simulink model "Hector"  (R2023b)
settings: Solver=daessc  StartTime=0.0  StopTime=1  FixedStep=0.001  MaxStep=1e-3  RelTol=1e-2
model workspace (MATLAB code in the model file):
  | %% World Plane
  | plane_x = 20;
  | plane_y = 2;
  | plane_z = 0.05;
  | 
  | %% motor
  | %A1
  | motor_com = [0, -0.02,0];
  | motor_com_mirror = [0, 0.02,0];
  | 
  | motor_I = [0.00048,0.00071,0.00048];
  | motor_mass = 0.605;
  | 
  | %% Body
  | % Inertial
  | body_com_x = 0.0;
  | body_com_y = 0.0;
  | body_com_z = -0.0;
  | body_mass = 5.75;
  | body_ixx = 44350*1e-6;
  | body_ixy = 0.0;
  | body_ixz = 0.0;
  | body_iyy = 53149*1e-6;
  | body_iyz = 0.0;
  | body_izz = 21390*1e-6;
  | 
  | %% Hip 1
  | % joint
  | hip1_offset_x =0.0;
  | hip1_offset_y = 0.047;
  | hip1_offset_z = 0.1265;
  | % hip1_max = 15;
  | % hip1_min = -15;
  | hip1_velocity_max = 21;
  | hip1_torque_max = 33.5;
  | % Inertial
  | hip1_com_x = 0.0268;
  | hip1_com_y = -0.00315;
  | hip1_com_z = -0.0272;
  | hip1_mass = 0.173;
  | hip1_ixx = 0.00022;
  | hip1_ixy = 0.0;
  | hip1_ixz = 0.0;
  | hip1_iyy = 0.00024;
  | hip1_iyz = 0.0;
  | hip1_izz = 0.00016;
  | 
  | %% Hip 2
  | % joint
  | hip2_offset_x =0.053;
  | hip2_offset_y = 0.0185;
  | hip2_offset_z = 0.071;
  | % hip2_max = 15;
  | % hip2_min = -15;
  | hip2_velocity_max = 21;
  | hip2_torque_max = 33.5;
  | % Inertial
  | hip2_com_x = -0.0308;
  | hip2_com_y = -0.00942;
  | hip2_com_z = 0.0;
  | hip2_mass = 0.0722;
  | hip2_ixx = 0.0000422;
  | hip2_ixy = 0.0;
  | hip2_ixz = 0.0;
  | hip2_iyy = 0.000120;
  | hip2_iyz = 0.0;
  | hip2_izz = 0.0000708;
  | 
  | %% Thigh
  | % joint
  | thigh_offset_x =-0.06;
  | thigh_offset_y = 0.004;
  | thigh_offset_z = 0.0;
  | % thigh_max = 130;
  | % thigh_min = -45;
  | thigh_velocity_max = 21;
  | thigh_torque_max = 33.5;
  | % Inertial
  | thigh_com_x = -0.00143;
  | thigh_com_y = -0.02106;
  | thigh_com_z = -0.06115;
  | thigh_mass = 0.397;
  | thigh_ixx = 0.00197;
  | thigh_ixy = 0.0;
  | thigh_ixz = 0.0;
  | thigh_iyy = 0.00218;
  | thigh_iyz = 0.0;
  | thigh_izz = 0.00033;
  | 
  | ankle_motor_offset_x = 0;
  | ankle_motor_offset_y = 0.039;
  | ankle_motor_offset_z = 0;
  | 
  | knee_motor_offset_x = 0;
  | knee_motor_offset_y = 0.039;
  | knee_motor_offset_z = -0.095;
  | 
  | %% Calf
  | % joint
  | calf_offset_x = 0.0;
  | calf_offset_y = 0.003;
  | calf_offset_z = -0.22;
  | % calf_max = 0;
  | % calf_min = -135;
  | % knee_max = 0;
  | % knee_min = -160;
  | calf_velocity_max = 14*1.5;
  | calf_torque_max = 51;
  | % Inertial
  | calf_com_x = 0.00165;
  | calf_com_y = -0.01117;
  | calf_com_z = -0.06438;
  | calf_mass = 0.136;
  | calf_ixx = 0.00071;
  | calf_ixy = 0.0;
  | calf_ixz = 0.0;
  | calf_iyy = 0.00072;
  | calf_iyz = 0.0;
  | calf_izz = 0.00002;
  | 
  | %% Toe
  | % joint
  | toe_offset_x = 0.0;
  | toe_offset_y = 0.011;
  | toe_offset_z = -0.22;
  | % toe_max = 60;
  | % toe_min = -60;
  | toe_velocity_max = 21;
  | toe_torque_max = 33.5;
  | % Inertial
  | toe_com_x = 0.00239;
  | toe_com_y = 0.00002;
  | toe_com_z = -0.02261;
  | toe_mass = 0.08425;
  | toe_ixx = 0.00001;
  | toe_ixy = 0.0;
  | toe_ixz = 0.0;
  | toe_iyy = 0.00011;
  | toe_iyz = 0.0;
  | toe_izz = 0.00011;
  | %% Contact
  | contact_front = 0.091;
  | contact_rear = -0.061;
  | contact_right = 0.026;
  | contact_left = 0.01;
  | contact_z = 0.039;
  | 
  | %%
  | %dorito
  | dorito_offset_x = 0;
  | dorito_offset_y = 0.012;
  | dorito_offset_z = 0;
  | 
  | dorito_lower_connection = [0.034 0 -0.044];
  | dorito_upper_connection = [0.034 0 0.021];
  | 
  | linkage_mass = 0.051;
  | linkage_com = [0 0 -0.11];
  | linkage_I = [0.00001 0.00002 0.00002];
  | %% Arms
  | shoulder_com_x = 0;
  | shoulder_com_y = 0;
  | shoulder_com_z = 0;
  | shoulder_mass = 0.835;
  | % shoulder_mass = 0.05;
  | shoulder_ixx = 920*1e-6;
  | shoulder_ixy = 0.0;
  | shoulder_ixz = 0.0;
  | shoulder_iyy = 270*1e-6;
  | shoulder_iyz = 0.0;
  | shoulder_izz = 499*1e-6;
  | 
  | upperarm_com_x = 0;
  | upperarm_com_y = 0;
  | upperarm_com_z = 0;
  | upperarm_mass = 1.35;
  | % upperarm_mass = 0.05;
  | upperarm_ixx = 1200*1e-6;
  | upperarm_ixy = 0.0;
  | upperarm_ixz = 0.0;
  | upperarm_iyy = 1170*1e-6;
  | upperarm_iyz = 0.0;
  | upperarm_izz = 729*1e-6;
  | 
  | forearm_com_x = 0;
  | forearm_com_y = 0;
  | forearm_com_z = -0.10;
  | forearm_mass = 0.53;
  | % forearm_mass = 0.03;
  | forearm_ixx = 427*1e-6;
  | forearm_ixy = 0.0;
  | forearm_ixz = 0.0;
  | forearm_iyy = 466*1e-6;
  | forearm_iyz = 0.0;
  | forearm_izz = 72*1e-6;
values from neighbouring files (symbols this model uses):
  body_v0 = [0 0 0]    [Initiate_Simulation.m]
  body_z0 = 0.55    [Initiate_Simulation.m]
  dt_MPC = gaitcycle/10    (= 0.04)    [Initiate_Simulation.m]
  N = 5000    [Initiate_Simulation.m]
  shoulderx_max = 90    [Initiate_Simulation.m]
  shoulderx_min = -15    [Initiate_Simulation.m]
  shoulderx_q0 = 0    [Initiate_Simulation.m]
undefined symbols (not defined in the file or in its folder): AssignMPCStage, sigbuilder_block, X, Y, Z
libraries: sm_lib x169, nesl_utility x95, dspindex x1, simulink x1
(part 5 of 7)

== system Hector/Hector/Left Leg/calf ==
  Joint : Inport
  Knee Joint : Subsystem
      settings: PortSchema="{\"entries\":[{\"content\":{\"sides\":[{\"content\":{\"connectorIds\":[\"LConn1\",\"In1\"]},\"type\":\"ConnectorPlacement.EquallySpacedRectSide\",\"uuid\":\"fe1bafd1-c1a5-4148-b465-5de294b235b8\"},{\"content\":{\"connectorIds\":[\"RConn1\",\"Out1\",\"Out2\",\"Out3\"],\"side\":\"RIGHT\"},\"type\":\"ConnectorPlacement.EquallySpacedRectSide\",\"uuid\":\"cbba8e06-0841-4611-b08d-047237296da9\"},{\"content\":{\"connectorIds\":[],\"side\":\"TOP\"},\"type\":\"ConnectorPlacement.EquallySpacedRectSide\",\"uuid\":\"b5035594-e8f7-4741-b410-9cfafd0751b0\"}]},\"type\":\"ConnectorPlacement.EquallySpacedConnector\",\"uuid\":\"2233606c-74e6-45bf-8a73-f401921fd730\"}],\"packageUris\":[\"http://schema.mathworks.com/mf0/Connector/R2020b\"],\"version\":\"1.0\"}"
  Rigid Transform4 : sm_lib/Frames and Transforms/Rigid Transform  TranslationMethod=None  TranslationStandardOffset=0  TranslationStandardOffsetUnits=m  TranslationStandardAxis=+Z  TranslationCartesianOffset=[0 0 0]  TranslationCartesianOffsetUnits=m  TranslationROffset=0  TranslationROffsetUnits=m  TranslationZOffset=0  TranslationZOffsetUnits=m  TranslationThetaOffset=0  TranslationThetaOffsetUnits=deg  RotationMethod=StandardAxis  RotationAngleUnits=deg  RotationStandardAxis=-X  RotationAngle=90  RotationArbitraryAxis=[0 0 1]  FollAlignAxisA=+X  BaseAlignAxisA=+Y  FollAlignAxisB=+Y  BaseAlignAxisB=+Z  RotationSequenceAxes=FollowerAxes  RotationSequence=XYX  RotationSequenceAngles=[0 0 0]  RotationSequenceAnglesUnits=deg  RotationMatrix=[1 0 0; 0 1 0; 0 0 1]  Quaternion=[1 0 0 0]
  Rigid Transform5 : sm_lib/Frames and Transforms/Rigid Transform  TranslationMethod=None  TranslationStandardOffset=0  TranslationStandardOffsetUnits=m  TranslationStandardAxis=+Z  TranslationCartesianOffset=[0 0 0]  TranslationCartesianOffsetUnits=m  TranslationROffset=0  TranslationROffsetUnits=m  TranslationZOffset=0  TranslationZOffsetUnits=m  TranslationThetaOffset=0  TranslationThetaOffsetUnits=deg  RotationMethod=StandardAxis  RotationAngleUnits=deg  RotationStandardAxis=+X  RotationAngle=90  RotationArbitraryAxis=[0 0 1]  FollAlignAxisA=+X  BaseAlignAxisA=+Y  FollAlignAxisB=+Y  BaseAlignAxisB=+Z  RotationSequenceAxes=FollowerAxes  RotationSequence=XYX  RotationSequenceAngles=[0 0 0]  RotationSequenceAnglesUnits=deg  RotationMatrix=[1 0 0; 0 1 0; 0 0 1]  Quaternion=[1 0 0 0]
  calf : sm_lib/Body Elements/File Solid  ExtGeomFileName=STL files\L_calf.STL  UnitType=Custom  ExtGeomFileUnits=m  StepReaderType=HEX  ExportConvexHullGeometry=off  InertiaType=Custom  Mass=calf_mass  MassUnits=kg  CenterOfMass=[calf_com_x -calf_com_y calf_com_z]  CenterOfMassUnits=m  MomentsOfInertia=[calf_ixx calf_iyy calf_izz]  MomentsOfInertiaUnits=kg*m^2  ProductsOfInertia=[0 0 0]  ProductsOfInertiaUnits=kg*m^2  BasedOnType=Density  Density=1000  DensityUnits=kg/m^3  DoExposeReferenceFrame=on  SerializedFrames=<Frames/>  GraphicType=FromGeometry  MarkerShape=Sphere  MarkerSize=10  GraphicVisPropType=AdvancedVisualProperties  GraphicDiffuseColor=[0.9 0.9 0.9]  GraphicSpecularColor=[0.7 0.7 0.7 1.0]  GraphicAmbientColor=[0.35 0.35 0.35 1.0]  GraphicEmissiveColor=[0.0 0.0 0.0 1.0]  GraphicShininess=5  GraphicOpacity=1.0
  B : PMIOPort  Side=Left
  Conn2 : PMIOPort  Port=2  Side=Right
  Sensor : Outport
  knee_angle : Outport  Port=2
  knee_angle_speed : Outport  Port=3
  wires:
  Knee Joint/2(knee_angle) -> knee_angle/1
  Knee Joint/3(knee_angle_speed) -> knee_angle_speed/1
  Knee Joint/1(Sensor) -> Sensor/1
  Joint/1 -> Knee Joint/1(Joint)
  connections:
  calf/RConn1 -- Rigid Transform4/LConn1
  Knee Joint/LConn1 -- B/RConn1
  Rigid Transform5/LConn1 -- Knee Joint/RConn1 -- Rigid Transform4/RConn1
  Rigid Transform5/RConn1 -- Conn2/RConn1

== system Hector/Hector/Left Leg/foot ==
  input : Inport
  Ankle Joint : Subsystem
      settings: PortSchema="{\"entries\":[{\"content\":{\"sides\":[{\"content\":{\"connectorIds\":[\"LConn1\",\"In1\"]},\"type\":\"ConnectorPlacement.EquallySpacedRectSide\",\"uuid\":\"d1094410-d7e2-420f-9299-c6db7682fd14\"},{\"content\":{\"connectorIds\":[\"RConn1\",\"Out1\"],\"side\":\"RIGHT\"},\"type\":\"ConnectorPlacement.EquallySpacedRectSide\",\"uuid\":\"17ca1f8d-2ad9-48dc-a054-4cdfe8b39b0e\"},{\"content\":{\"side\":\"TOP\"},\"type\":\"ConnectorPlacement.EquallySpacedRectSide\",\"uuid\":\"c0a1fb68-cc05-4666-9aff-395b76c49866\"}]},\"type\":\"ConnectorPlacement.EquallySpacedConnector\",\"uuid\":\"a0ca8f3e-9cc5-4e2d-aebb-075ea702600d\"}],\"packageUris\":[\"http://schema.mathworks.com/mf0/Connector/R2020b\"],\"version\":\"1.0\"}"
  Foot : sm_lib/Body Elements/File Solid  ExtGeomFileName=STL files\L_foot.STL  UnitType=Custom  ExtGeomFileUnits=m  StepReaderType=HEX  ExportConvexHullGeometry=off  InertiaType=Custom  Mass=toe_mass  MassUnits=kg  CenterOfMass=[toe_com_x toe_com_y toe_com_z]  CenterOfMassUnits=m  MomentsOfInertia=[toe_ixx toe_iyy toe_izz]  MomentsOfInertiaUnits=kg*m^2  ProductsOfInertia=[0 0 0]  ProductsOfInertiaUnits=kg*m^2  BasedOnType=Density  Density=1000  DensityUnits=kg/m^3  DoExposeReferenceFrame=on  SerializedFrames=<Frames/>  GraphicType=FromGeometry  MarkerShape=Sphere  MarkerSize=10  GraphicVisPropType=AdvancedVisualProperties  GraphicDiffuseColor=[0.9 0.9 0.9]  GraphicSpecularColor=[0.7 0.7 0.7 1.0]  GraphicAmbientColor=[0.35 0.35 0.35 1.0]  GraphicEmissiveColor=[0.0 0.0 0.0 1.0]  GraphicShininess=5  GraphicOpacity=1.0
  Rigid Transform1 : sm_lib/Frames and Transforms/Rigid Transform  TranslationMethod=Cartesian  TranslationStandardOffset=0  TranslationStandardOffsetUnits=m  TranslationStandardAxis=+Z  TranslationCartesianOffset=[0 0.01 0]  TranslationCartesianOffsetUnits=m  TranslationROffset=0  TranslationROffsetUnits=m  TranslationZOffset=0  TranslationZOffsetUnits=m  TranslationThetaOffset=0  TranslationThetaOffsetUnits=deg  RotationMethod=None  RotationAngleUnits=deg  RotationStandardAxis=-X  RotationAngle=90  RotationArbitraryAxis=[0 0 1]  FollAlignAxisA=+X  BaseAlignAxisA=+Y  FollAlignAxisB=+Y  BaseAlignAxisB=+Z  RotationSequenceAxes=FollowerAxes  RotationSequence=XYX  RotationSequenceAngles=[0 0 0]  RotationSequenceAnglesUnits=deg  RotationMatrix=[1 0 0; 0 1 0; 0 0 1]  Quaternion=[1 0 0 0]
  Rigid Transform6 : sm_lib/Frames and Transforms/Rigid Transform  TranslationMethod=None  TranslationStandardOffset=0  TranslationStandardOffsetUnits=m  TranslationStandardAxis=+Z  TranslationCartesianOffset=[0 0 0]  TranslationCartesianOffsetUnits=m  TranslationROffset=0  TranslationROffsetUnits=m  TranslationZOffset=0  TranslationZOffsetUnits=m  TranslationThetaOffset=0  TranslationThetaOffsetUnits=deg  RotationMethod=StandardAxis  RotationAngleUnits=deg  RotationStandardAxis=-X  RotationAngle=90  RotationArbitraryAxis=[0 0 1]  FollAlignAxisA=+X  BaseAlignAxisA=+Y  FollAlignAxisB=+Y  BaseAlignAxisB=+Z  RotationSequenceAxes=FollowerAxes  RotationSequence=XYX  RotationSequenceAngles=[0 0 0]  RotationSequenceAnglesUnits=deg  RotationMatrix=[1 0 0; 0 1 0; 0 0 1]  Quaternion=[1 0 0 0]
  B : PMIOPort  Side=Left
  Conn4 : PMIOPort  Port=2  Side=Right
  F : PMIOPort  Port=3  Side=Right
  sensor : Outport
  wires:
  input/1 -> Ankle Joint/1(input)
  Ankle Joint/1(sensor) -> sensor/1
  connections:
  Rigid Transform6/RConn1 -- Ankle Joint/RConn1
  Ankle Joint/LConn1 -- B/RConn1
  Rigid Transform6/LConn1 -- Conn4/RConn1 -- Rigid Transform1/RConn1 -- F/RConn1
  Rigid Transform1/LConn1 -- Foot/RConn1

== system Hector/Hector/Left Leg/hip location sensor ==
  Bus Creator : BusCreator  Inputs=3
  PS-Simulink Converter : nesl_utility/PS-Simulink Converter  PhysicalDomain=network_engine_domain  SubClassName=ps_output  LeftPortType=input  RightPortType=output  PseudoPeriodic=off  Frequencies=[]  VectorFormat=1-D array  Unit=inherit  AffineConversion=off
  PS-Simulink Converter1 : nesl_utility/PS-Simulink Converter  PhysicalDomain=network_engine_domain  SubClassName=ps_output  LeftPortType=input  RightPortType=output  PseudoPeriodic=off  Frequencies=[]  VectorFormat=1-D array  Unit=inherit  AffineConversion=off
  PS-Simulink Converter2 : nesl_utility/PS-Simulink Converter  PhysicalDomain=network_engine_domain  SubClassName=ps_output  LeftPortType=input  RightPortType=output  PseudoPeriodic=off  Frequencies=[]  VectorFormat=1-D array  Unit=inherit  AffineConversion=off
  Transform Sensor : sm_lib/Frames and Transforms/Transform Sensor  MeasurementFrame=World  RotationSequence=XYX  SenseAngle=off  SenseAxis=off  SenseQ=off  SenseR=off  SenseRotationSequence=off  SenseOmegaX=off  SenseOmegaY=off  SenseOmegaZ=off  SenseOmega=off  SenseQDot=off  SenseRDot=off  SenseRotationSequenceDot=off  SenseAlphaX=off  SenseAlphaY=off  SenseAlphaZ=off  SenseAlpha=off  SenseQDDot=off  SenseRDDot=off  SenseX=on  SenseY=on  SenseZ=on  SenseXYZ=off  SenseRad=off  SenseAzim=off  SenseDist=off  SenseInc=off  SenseXDot=off  SenseYDot=off  SenseZDot=off  SenseXYZDot=off  SenseRadDot=off  SenseAzimDot=off  SenseDistDot=off  SenseIncDot=off  SenseXDDot=off  SenseYDDot=off  SenseZDDot=off  SenseXYZDDot=off  SenseRadDDot=off  SenseAzimDDot=off  SenseDistDDot=off  SenseIncDDot=off
  World Frame : sm_lib/Frames and Transforms/World Frame
  R : PMIOPort  Side=Right
  hip_location : Outport
  wires:
  PS-Simulink Converter1/1 -> Bus Creator/2  "y"
  PS-Simulink Converter/1 -> Bus Creator/1  "x"
  PS-Simulink Converter2/1 -> Bus Creator/3  "z"
  Bus Creator/1 -> hip_location/1
  connections:
  PS-Simulink Converter2/LConn1 -- Transform Sensor/RConn4
  PS-Simulink Converter/LConn1 -- Transform Sensor/RConn2
  World Frame/RConn1 -- Transform Sensor/LConn1
  PS-Simulink Converter1/LConn1 -- Transform Sensor/RConn3
  Transform Sensor/RConn1 -- R/RConn1

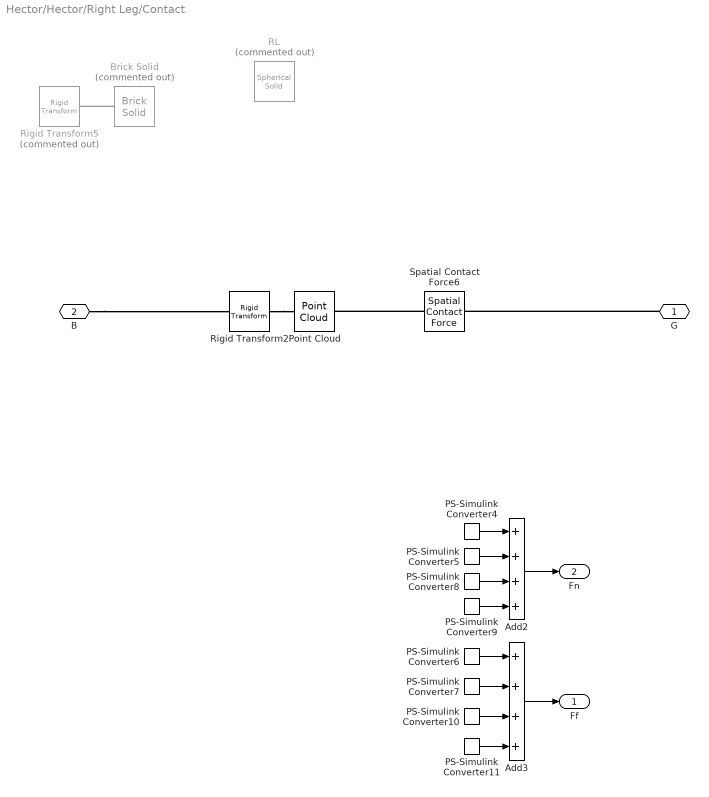
== system Hector/Hector/Right Leg/Contact ==
  Add2 : Sum  Inputs=++++
  Add3 : Sum  Inputs=++++
  Brick Solid : sm_lib/Body Elements/Brick Solid  Commented=on  GraphicAmbientColor=[0.15 0.15 0.15 1.0]  BasedOnType=Density  BrickDimensions=[0.16 0.02 0.0001]  BrickDimensionsUnits=m  CenterOfMass=[0 0 0]  CenterOfMassUnits=m  GraphicDiffuseColor=[0.5 0.5 0.5]  Density=1000  DensityUnits=kg/m^3  DoExposeReferenceFrame=on  GraphicEmissiveColor=[0.0 0.0 0.0 1.0]  ExportEntireGeometry=on  SerializedFrames=<Frames/>  MarkerShape=Sphere  MarkerSize=10  GraphicType=FromGeometry  InertiaType=PointMass  Mass=0  MassUnits=kg  MomentsOfInertia=[1 1 1]  MomentsOfInertiaUnits=kg*m^2  GraphicOpacity=1.0  ProductsOfInertia=[0 0 0]  ProductsOfInertiaUnits=kg*m^2  GraphicShininess=75  GraphicSpecularColor=[0.5 0.5 0.5 1.0]  GraphicVisPropType=SimpleVisualProperties
  PS-Simulink Converter{4..11} (8 alike) : nesl_utility/PS-Simulink Converter  PhysicalDomain=network_engine_domain  SubClassName=ps_output  LeftPortType=input  RightPortType=output  PseudoPeriodic=off  Frequencies=[]  VectorFormat=1-D array  Unit=inherit  AffineConversion=off
  Point Cloud : sm_lib/Curves and Surfaces/Point Cloud  CoordinatesMatrix=contact_cloud  CoordinatesMatrixUnits=m  GraphicType=MarkerCloud  GraphicSphereRadius=0.001  GraphicSphereRadiusUnits=m  GraphicVisPropType=SimpleVisualProperties  GraphicDiffuseColor=[0.5 0.5 0.5]  GraphicOpacity=1.0  GraphicSpecularColor=[0.5 0.5 0.5 1.0]  GraphicAmbientColor=[0.15 0.15 0.15 1.0]  GraphicEmissiveColor=[0.0 0.0 0.0 1.0]  GraphicShininess=75
  RL : sm_lib/Body Elements/Spherical Solid  Commented=on  GraphicAmbientColor=[0.15 0.15 0.15 1.0]  BasedOnType=Density  CenterOfMass=[0 0 0]  CenterOfMassUnits=m  GraphicDiffuseColor=[1.0 0.0 0.2]  Density=0  DensityUnits=kg/m^3  DoExposeReferenceFrame=on  GraphicEmissiveColor=[0.0 0.0 0.0 1.0]  ExportEntireGeometry=on  SerializedExposedGeometries=<ExposedGeometries><ExposedGeometry><RawGeometryId>entire</RawGeometryId><ExposedGeometryId>G</ExposedGeometryId></ExposedGeometry></ExposedGeometries>  SerializedFrames=<Frames/>  MarkerShape=Sphere  MarkerSize=10  GraphicType=FromGeometry  InertiaType=CalculateFromGeometry  Mass=1  MassUnits=kg  MomentsOfInertia=[1 1 1]  MomentsOfInertiaUnits=kg*m^2  GraphicOpacity=1.0  ProductsOfInertia=[0 0 0]  ProductsOfInertiaUnits=kg*m^2  GraphicShininess=75  GraphicSpecularColor=[0.5 0.5 0.5 1.0]  SphereRadius=contact_point_radius  SphereRadiusUnits=m  GraphicVisPropType=SimpleVisualProperties
  Rigid Transform2 : sm_lib/Frames and Transforms/Rigid Transform  TranslationMethod=Cartesian  TranslationStandardOffset=0  TranslationStandardOffsetUnits=m  TranslationStandardAxis=+Z  TranslationCartesianOffset=[0 0.0 -contact_z]  TranslationCartesianOffsetUnits=m  TranslationROffset=0  TranslationROffsetUnits=m  TranslationZOffset=0  TranslationZOffsetUnits=m  TranslationThetaOffset=0  TranslationThetaOffsetUnits=deg  RotationMethod=None  RotationAngleUnits=deg  RotationStandardAxis=+Z  RotationAngle=0.0  RotationArbitraryAxis=[0 0 1]  FollAlignAxisA=+X  BaseAlignAxisA=+Y  FollAlignAxisB=+Y  BaseAlignAxisB=+Z  RotationSequenceAxes=FollowerAxes  RotationSequence=XYX  RotationSequenceAngles=[0 0 0]  RotationSequenceAnglesUnits=deg  RotationMatrix=[1 0 0; 0 1 0; 0 0 1]  Quaternion=[1 0 0 0]
  Rigid Transform5 : sm_lib/Frames and Transforms/Rigid Transform  Commented=on  TranslationMethod=Cartesian  TranslationStandardOffset=0  TranslationStandardOffsetUnits=m  TranslationStandardAxis=+Z  TranslationCartesianOffset=[0.015 2*contact_left -contact_z]  TranslationCartesianOffsetUnits=m  TranslationROffset=0  TranslationROffsetUnits=m  TranslationZOffset=0  TranslationZOffsetUnits=m  TranslationThetaOffset=0  TranslationThetaOffsetUnits=deg  RotationMethod=None  RotationAngleUnits=deg  RotationStandardAxis=+Z  RotationAngle=0.0  RotationArbitraryAxis=[0 0 1]  FollAlignAxisA=+X  BaseAlignAxisA=+Y  FollAlignAxisB=+Y  BaseAlignAxisB=+Z  RotationSequenceAxes=FollowerAxes  RotationSequence=XYX  RotationSequenceAngles=[0 0 0]  RotationSequenceAnglesUnits=deg  RotationMatrix=[1 0 0; 0 1 0; 0 0 1]  Quaternion=[1 0 0 0]
  Spatial Contact Force6 : sm_lib/Forces and Torques/Spatial Contact Force  SenseContactBaseRotation=off  SenseContactBaseTranslation=off  CoefficientOfDynamicFriction=mu_k  CoefficientOfStaticFriction=mu_s  NormalDamping=contact_damping  NormalDampingUnits=N/(m/s)  SenseContactSignal=off  NormalStiffness=contact_stiffness  NormalStiffnessUnits=N/m  FrictionalCriticalVelocity=mu_vth  FrictionalCriticalVelocityUnits=m/s  ZeroCrossDetectContactStartAndEnd=off  SenseContactFollowerRotation=off  SenseContactFollowerTranslation=off  FrictionType=SmoothStickSlip  SenseFrictionalForceMagnitude=off  SenseNormalForceMagnitude=off  NormalForceType=SmoothSpringDamper  SenseNormalVelocity=off  SensePenetrationDepth=off  SenseSeparationDistance=off  SenseTangentialVelocity=off  NormalTransitionRegionWidth=1e-4  NormalTransitionRegionWidthUnits=m
  G : PMIOPort  Side=Left
  B : PMIOPort  Port=2  Side=Right
  Ff : Outport
  Fn : Outport  Port=2
  wires:
  PS-Simulink Converter11/1 -> Add3/4
  PS-Simulink Converter9/1 -> Add2/4
  PS-Simulink Converter8/1 -> Add2/3
  PS-Simulink Converter5/1 -> Add2/2
  PS-Simulink Converter6/1 -> Add3/1
  Add2/1 -> Fn/1
  PS-Simulink Converter4/1 -> Add2/1
  PS-Simulink Converter10/1 -> Add3/3
  Add3/1 -> Ff/1
  PS-Simulink Converter7/1 -> Add3/2
  connections:
  G/RConn1 -- Spatial Contact Force6/LConn1
  Brick Solid/RConn1 -- Rigid Transform5/RConn1
  Spatial Contact Force6/RConn1 -- Point Cloud/RConn1
  B/RConn1 -- Rigid Transform2/LConn1
  Rigid Transform2/RConn1 -- Point Cloud/LConn1

== system Hector/Hector/Right Leg/Hip Roll  ==
  joint : Inport
  Hip 2 : sm_lib/Body Elements/File Solid  ExtGeomFileName=STL files\R_hip2.STL  UnitType=Custom  ExtGeomFileUnits=m  StepReaderType=HEX  ExportConvexHullGeometry=off  InertiaType=Custom  Mass=hip2_mass  MassUnits=kg  CenterOfMass=[hip2_com_x hip2_com_y hip2_com_z]  CenterOfMassUnits=m  MomentsOfInertia=[hip2_ixx hip2_iyy hip2_izz]  MomentsOfInertiaUnits=kg*m^2  ProductsOfInertia=[0 0 0]  ProductsOfInertiaUnits=kg*m^2  BasedOnType=Density  Density=1000  DensityUnits=kg/m^3  DoExposeReferenceFrame=on  SerializedFrames=<Frames/>  GraphicType=FromGeometry  MarkerShape=Sphere  MarkerSize=10  GraphicVisPropType=AdvancedVisualProperties  GraphicDiffuseColor=[0.9 0.9 0.9]  GraphicSpecularColor=[0.7 0.7 0.7 1.0]  GraphicAmbientColor=[0.35 0.35 0.35 1.0]  GraphicEmissiveColor=[0.0 0.0 0.0 1.0]  GraphicShininess=5  GraphicOpacity=1.0
  Hip Roll Joint : Subsystem
      settings: PortSchema="{\"entries\":[{\"content\":{\"sides\":[{\"content\":{\"connectorIds\":[\"LConn1\",\"In1\"]},\"type\":\"ConnectorPlacement.EquallySpacedRectSide\",\"uuid\":\"fe1bafd1-c1a5-4148-b465-5de294b235b8\"},{\"content\":{\"connectorIds\":[\"RConn1\",\"Out1\"],\"side\":\"RIGHT\"},\"type\":\"ConnectorPlacement.EquallySpacedRectSide\",\"uuid\":\"cbba8e06-0841-4611-b08d-047237296da9\"},{\"content\":{\"connectorIds\":[],\"side\":\"TOP\"},\"type\":\"ConnectorPlacement.EquallySpacedRectSide\",\"uuid\":\"b5035594-e8f7-4741-b410-9cfafd0751b0\"}]},\"type\":\"ConnectorPlacement.EquallySpacedConnector\",\"uuid\":\"2233606c-74e6-45bf-8a73-f401921fd730\"}],\"packageUris\":[\"http://schema.mathworks.com/mf0/Connector/R2020b\"],\"version\":\"1.0\"}"
  Rigid Transform : sm_lib/Frames and Transforms/Rigid Transform  TranslationMethod=None  TranslationStandardOffset=0  TranslationStandardOffsetUnits=m  TranslationStandardAxis=+Z  TranslationCartesianOffset=[0 0 0]  TranslationCartesianOffsetUnits=m  TranslationROffset=0  TranslationROffsetUnits=m  TranslationZOffset=0  TranslationZOffsetUnits=m  TranslationThetaOffset=0  TranslationThetaOffsetUnits=deg  RotationMethod=StandardAxis  RotationAngleUnits=deg  RotationStandardAxis=+Y  RotationAngle=90  RotationArbitraryAxis=[0 0 1]  FollAlignAxisA=+X  BaseAlignAxisA=+Y  FollAlignAxisB=+Y  BaseAlignAxisB=+Z  RotationSequenceAxes=FollowerAxes  RotationSequence=XYX  RotationSequenceAngles=[0 0 0]  RotationSequenceAnglesUnits=deg  RotationMatrix=[1 0 0; 0 1 0; 0 0 1]  Quaternion=[1 0 0 0]
  Rigid Transform1 : sm_lib/Frames and Transforms/Rigid Transform  TranslationMethod=None  TranslationStandardOffset=0  TranslationStandardOffsetUnits=m  TranslationStandardAxis=+Z  TranslationCartesianOffset=[0 0 0]  TranslationCartesianOffsetUnits=m  TranslationROffset=0  TranslationROffsetUnits=m  TranslationZOffset=0  TranslationZOffsetUnits=m  TranslationThetaOffset=0  TranslationThetaOffsetUnits=deg  RotationMethod=StandardAxis  RotationAngleUnits=deg  RotationStandardAxis=+Y  RotationAngle=-90  RotationArbitraryAxis=[0 0 1]  FollAlignAxisA=+X  BaseAlignAxisA=+Y  FollAlignAxisB=+Y  BaseAlignAxisB=+Z  RotationSequenceAxes=FollowerAxes  RotationSequence=XYX  RotationSequenceAngles=[0 0 0]  RotationSequenceAnglesUnits=deg  RotationMatrix=[1 0 0; 0 1 0; 0 0 1]  Quaternion=[1 0 0 0]
  Rigid Transform2 : sm_lib/Frames and Transforms/Rigid Transform  TranslationMethod=Cartesian  TranslationStandardOffset=0  TranslationStandardOffsetUnits=m  TranslationStandardAxis=+Z  TranslationCartesianOffset=[thigh_offset_x -thigh_offset_y -thigh_offset_z]  TranslationCartesianOffsetUnits=m  TranslationROffset=0  TranslationROffsetUnits=m  TranslationZOffset=0  TranslationZOffsetUnits=m  TranslationThetaOffset=0  TranslationThetaOffsetUnits=deg  RotationMethod=None  RotationAngleUnits=deg  RotationStandardAxis=+Z  RotationAngle=90  RotationArbitraryAxis=[0 0 1]  FollAlignAxisA=+X  BaseAlignAxisA=+Y  FollAlignAxisB=+Y  BaseAlignAxisB=+Z  RotationSequenceAxes=FollowerAxes  RotationSequence=XYX  RotationSequenceAngles=[0 0 0]  RotationSequenceAnglesUnits=deg  RotationMatrix=[1 0 0; 0 1 0; 0 0 1]  Quaternion=[1 0 0 0]
  motor : sm_lib/Body Elements/File Solid  ExtGeomFileName=STL files/A1motor_mirror.STL  UnitType=Custom  ExtGeomFileUnits=m  StepReaderType=HEX  ExportConvexHullGeometry=off  InertiaType=Custom  Mass=0.605  MassUnits=kg  CenterOfMass=motor_com_mirror  CenterOfMassUnits=m  MomentsOfInertia=motor_I  MomentsOfInertiaUnits=kg*m^2  ProductsOfInertia=[0 0 0]  ProductsOfInertiaUnits=kg*m^2  BasedOnType=DensityFromFile  Density=1000  DensityUnits=kg/m^3  DoExposeReferenceFrame=on  SerializedFrames=<Frames/>  GraphicType=FromGeometry  MarkerShape=Sphere  MarkerSize=10  GraphicVisPropType=SimpleVisualProperties  GraphicDiffuseColor=[0.2 0.2 0.2]  GraphicSpecularColor=[0.5 0.5 0.5 1.0]  GraphicAmbientColor=[0.15 0.15 0.15 1.0]  GraphicEmissiveColor=[0.0 0.0 0.0 1.0]  GraphicShininess=75  GraphicOpacity=1.0
  B : PMIOPort  Side=Left
  F : PMIOPort  Port=2  Side=Right
  Sensor : Outport
  wires:
  Hip Roll Joint/1(Sensor) -> Sensor/1
  joint/1 -> Hip Roll Joint/1(joint)
  connections:
  Rigid Transform1/LConn1 -- Rigid Transform/RConn1 -- Hip Roll Joint/RConn1
  Hip Roll Joint/LConn1 -- B/RConn1
  F/RConn1 -- Rigid Transform1/RConn1
  Rigid Transform/LConn1 -- Hip 2/RConn1 -- Rigid Transform2/LConn1
  Rigid Transform2/RConn1 -- motor/RConn1

== system Hector/Hector/Right Leg/Hip Yaw  ==
  Joint : Inport
  Hip 1 : sm_lib/Body Elements/File Solid  ExtGeomFileName=STL files\R_hip1.STL  UnitType=Custom  ExtGeomFileUnits=m  StepReaderType=HEX  ExportConvexHullGeometry=off  InertiaType=Custom  Mass=hip1_mass  MassUnits=kg  CenterOfMass=[hip1_com_x hip1_com_y hip1_com_z]  CenterOfMassUnits=m  MomentsOfInertia=[hip1_ixx hip1_iyy hip1_izz]  MomentsOfInertiaUnits=kg*m^2  ProductsOfInertia=[0 0 0]  ProductsOfInertiaUnits=kg*m^2  BasedOnType=Density  Density=1000  DensityUnits=kg/m^3  DoExposeReferenceFrame=on  SerializedFrames=<Frames/>  GraphicType=FromGeometry  MarkerShape=Sphere  MarkerSize=10  GraphicVisPropType=AdvancedVisualProperties  GraphicDiffuseColor=[0.9 0.9 0.9]  GraphicSpecularColor=[0.7 0.7 0.7 1.0]  GraphicAmbientColor=[0.35 0.35 0.35 1.0]  GraphicEmissiveColor=[0.0 0.0 0.0 1.0]  GraphicShininess=5  GraphicOpacity=1.0
  Hip Yaw Joint : Subsystem
      settings: PortSchema="{\"entries\":[{\"content\":{\"sides\":[{\"content\":{\"connectorIds\":[\"LConn1\",\"In1\"]},\"type\":\"ConnectorPlacement.EquallySpacedRectSide\",\"uuid\":\"b3c964c5-c8eb-47b4-9e52-3baca431b477\"},{\"content\":{\"connectorIds\":[\"RConn1\",\"Out1\"],\"side\":\"RIGHT\"},\"type\":\"ConnectorPlacement.EquallySpacedRectSide\",\"uuid\":\"b5493eb8-f54f-4e30-9772-3f18358e11ff\"},{\"content\":{\"connectorIds\":[],\"side\":\"TOP\"},\"type\":\"ConnectorPlacement.EquallySpacedRectSide\",\"uuid\":\"48e308f5-e3ea-4422-818b-169dbf54879a\"}]},\"type\":\"ConnectorPlacement.EquallySpacedConnector\",\"uuid\":\"dc2c179e-5c3d-431a-a3fe-d4dab1fabc56\"}],\"packageUris\":[\"http://schema.mathworks.com/mf0/Connector/R2020b\"],\"version\":\"1.0\"}"
  Rigid Transform : sm_lib/Frames and Transforms/Rigid Transform  TranslationMethod=Cartesian  TranslationStandardOffset=0  TranslationStandardOffsetUnits=m  TranslationStandardAxis=+Z  TranslationCartesianOffset=[hip2_offset_x -hip2_offset_y -hip2_offset_z]  TranslationCartesianOffsetUnits=m  TranslationROffset=0  TranslationROffsetUnits=m  TranslationZOffset=0  TranslationZOffsetUnits=m  TranslationThetaOffset=0  TranslationThetaOffsetUnits=deg  RotationMethod=StandardAxis  RotationAngleUnits=deg  RotationStandardAxis=+Z  RotationAngle=90  RotationArbitraryAxis=[0 0 1]  FollAlignAxisA=+X  BaseAlignAxisA=+Y  FollAlignAxisB=+Y  BaseAlignAxisB=+Z  RotationSequenceAxes=FollowerAxes  RotationSequence=XYX  RotationSequenceAngles=[0 0 0]  RotationSequenceAnglesUnits=deg  RotationMatrix=[1 0 0; 0 1 0; 0 0 1]  Quaternion=[1 0 0 0]
  motor : sm_lib/Body Elements/File Solid  ExtGeomFileName=STL files/A1motor.STL  UnitType=Custom  ExtGeomFileUnits=m  StepReaderType=HEX  ExportConvexHullGeometry=off  InertiaType=Custom  Mass=0.605  MassUnits=kg  CenterOfMass=motor_com  CenterOfMassUnits=m  MomentsOfInertia=motor_I  MomentsOfInertiaUnits=kg*m^2  ProductsOfInertia=[0 0 0]  ProductsOfInertiaUnits=kg*m^2  BasedOnType=DensityFromFile  Density=1000  DensityUnits=kg/m^3  DoExposeReferenceFrame=on  SerializedFrames=<Frames/>  GraphicType=FromGeometry  MarkerShape=Sphere  MarkerSize=10  GraphicVisPropType=SimpleVisualProperties  GraphicDiffuseColor=[0.2 0.2 0.2]  GraphicSpecularColor=[0.5 0.5 0.5 1.0]  GraphicAmbientColor=[0.15 0.15 0.15 1.0]  GraphicEmissiveColor=[0.0 0.0 0.0 1.0]  GraphicShininess=75  GraphicOpacity=1.0
  B : PMIOPort  Side=Left
  F : PMIOPort  Port=2  Side=Right
  Sensor : Outport
  wires:
  Joint/1 -> Hip Yaw Joint/1(Joint)
  Hip Yaw Joint/1(Sensor) -> Sensor/1
  connections:
  Hip 1/RConn1 -- F/RConn1 -- Hip Yaw Joint/RConn1 -- Rigid Transform/LConn1
  Hip Yaw Joint/LConn1 -- B/RConn1
  Rigid Transform/RConn1 -- motor/RConn1
